simulink model "quadcopter_LQR_test"  (R2015b)
settings: Solver=VariableStepAuto  StartTime=0.0  StopTime=50  RelTol=1e-3
undefined symbols (not defined in the file or in its folder): g, K, k, m, omegalim, seed
libraries: vrlib x2
settings Model: Creator=Daniel  LastModifiedBy=mgreiff
settings SolverCC: AlgebraicLoopSolver=LineSearch

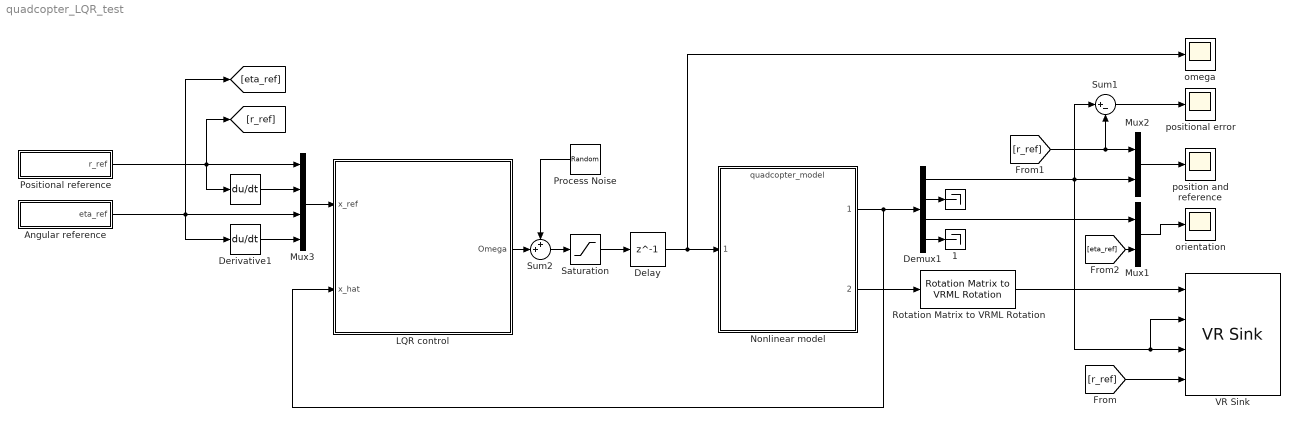
== system quadcopter_LQR_test ==
  "  " : Terminator
  "        " : Derivative
  "   1" : Terminator
  Angular reference : Subsystem
  Delay : Delay  DelayLength=1  InitialCondition=0  SampleTime=0.01
  Demux1 : Demux  Outputs=[3,3,3,3]
  Derivative1 : Derivative
  LQR control : Subsystem
  Mux1 : Mux  Inputs=2
  Mux2 : Mux  Inputs=2
  Mux3 : Mux  Inputs=[3,3,3,3]
  Nonlinear model : ModelReference  ModelNameDialog=quadcopter_model.mdl  SimulationMode=Normal  ModelReferenceVersion=1.117  CopyOfModelName=quadcopter_model.mdl
  Positional reference : Subsystem
  Process Noise : RandomNumber  Mean=[0 0 0 0]'  Variance=0  SampleTime=0.01
  Rotation Matrix to VRML Rotation : vrlib/Utilities/Rotation Matrix to VRML Rotation  maxzero=1e-12
  Saturation : Saturate  UpperLimit=omegalim(2)  LowerLimit=omegalim(1)
  Sum1 : Sum  Inputs=|+-
  Sum2 : Sum  Inputs=++|
  VR Sink : vrlib/VR Sink  InstantiateOnLoad=on  SampleTime=0.05  ViewEnable=on  RemoteChange=off  RemoteView=off  FieldsWritten=copter.rotation.4.1.1.double#copter.translation.3.1.1.double#vp.translation.3.1.1.double#target.translation.3.1.1.double  WorldFileName=copter_world.wrl  WorldDescription=quadcopter_world  AutoView=on  VideoDimensions=[]  AllowVariableSize=off
  "omega " : Scope
  orientation : Scope
  position and reference : Scope
  positional error : Scope
  wires:
  Saturation/1 -> Delay/1
  Nonlinear model/2 -> Rotation Matrix to VRML Rotation/1
  Rotation Matrix to VRML Rotation/1 -> VR Sink/1
  Process Noise/1 -> Sum2/1
  Sum2/1 -> Saturation/1
  Delay/1 -> "omega "/1, Nonlinear model/1
  LQR control/1(Omega) -> Sum2/2
  Angular reference/1(eta_ref) -> Derivative1/1, Mux3/3, [eta_ref]
  [r_ref] -> VR Sink/4
  Positional reference/1(r_ref) -> [r_ref], Mux3/1, "        "/1
  [r_ref] -> Sum1/2, Mux2/1
  Mux2/1 -> position and reference/1
  Sum1/1 -> positional error/1
  Demux1/1 -> VR Sink/2, VR Sink/3, Sum1/1, Mux2/2
  Demux1/2 -> "  "/1
  Demux1/4 -> "   1"/1
  Nonlinear model/1 -> LQR control/2(x_hat), Demux1/1
  Demux1/3 -> Mux1/1
  Mux1/1 -> orientation/1
  [eta_ref] -> Mux1/2
  "        "/1 -> Mux3/2
  Derivative1/1 -> Mux3/4
  Mux3/1 -> LQR control/1(x_ref)

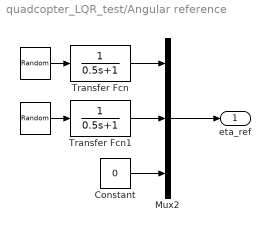
== system quadcopter_LQR_test/Angular reference ==
  " " : UniformRandomNumber  Minimum=-0.2  Maximum=0.2  Seed=4+seed  SampleTime=10
  "   " : UniformRandomNumber  Minimum=-0.2  Maximum=0.2  Seed=3+seed  SampleTime=10
  Constant : Constant  Value=0
  Mux2 : Mux  Inputs=3
  Transfer Fcn : TransferFcn  Denominator=[0.5 1]
  Transfer Fcn1 : TransferFcn  Denominator=[0.5 1]
  eta_ref : Outport
  wires:
  Mux2/1 -> eta_ref/1
  "   "/1 -> Transfer Fcn/1
  " "/1 -> Transfer Fcn1/1
  Transfer Fcn/1 -> Mux2/1
  Transfer Fcn1/1 -> Mux2/2
  Constant/1 -> Mux2/3

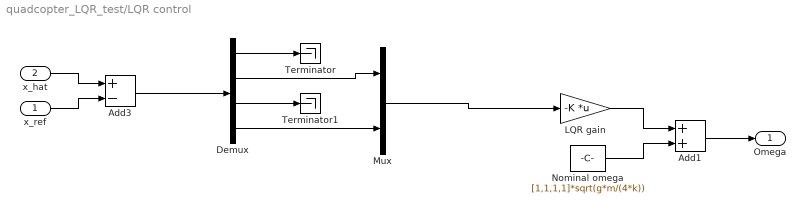
== system quadcopter_LQR_test/LQR control ==
  x_ref : Inport  PortDimensions=12
  x_hat : Inport  Port=2  PortDimensions=12
  Add1 : Sum
  Add3 : Sum  Inputs=+-
  Demux : Demux  Outputs=[2,1,2,7]
  LQR gain : Gain  Gain=-K  Multiplication=Matrix(K*u)
  Mux : Mux  Inputs=2
  Nominal omega : Constant  Value=[1,1,1,1]*sqrt(g*m/(4*k))
  Terminator : Terminator
  Terminator1 : Terminator
  Omega : Outport
  wires:
  Mux/1 -> LQR gain/1
  LQR gain/1 -> Add1/1
  Nominal omega/1 -> Add1/2
  Add1/1 -> Omega/1
  Demux/1 -> Terminator/1
  x_ref/1 -> Add3/2
  x_hat/1 -> Add3/1
  Add3/1 -> Demux/1
  Demux/2 -> Mux/1
  Demux/3 -> Terminator1/1
  Demux/4 -> Mux/2

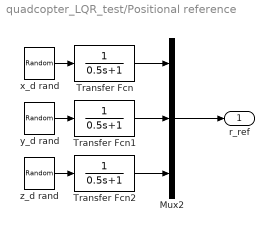
== system quadcopter_LQR_test/Positional reference ==
  Mux2 : Mux  Inputs=3
  Transfer Fcn : TransferFcn  Denominator=[0.5 1]
  Transfer Fcn1 : TransferFcn  Denominator=[0.5 1]
  Transfer Fcn2 : TransferFcn  Denominator=[0.5 1]
  x_d rand : UniformRandomNumber  Minimum=-30  Maximum=30  Seed=0+seed  SampleTime=10
  y_d rand : UniformRandomNumber  Minimum=-30  Maximum=30  Seed=1+seed  SampleTime=10
  z_d rand : UniformRandomNumber  Minimum=0  Maximum=15  Seed=2+seed  SampleTime=10
  r_ref : Outport
  wires:
  Mux2/1 -> r_ref/1
  x_d rand/1 -> Transfer Fcn/1
  y_d rand/1 -> Transfer Fcn1/1
  z_d rand/1 -> Transfer Fcn2/1
  Transfer Fcn/1 -> Mux2/1
  Transfer Fcn1/1 -> Mux2/2
  Transfer Fcn2/1 -> Mux2/3
